simulink model "front_observer"  (R2025b)
settings: Solver=VariableStepAuto  StartTime=0.0  StopTime=60  RelTol=1e-3
undefined symbols (not defined in the file): A, B, C, L
settings Model: Creator=lilkiddy  LastModifiedBy=lilkiddy

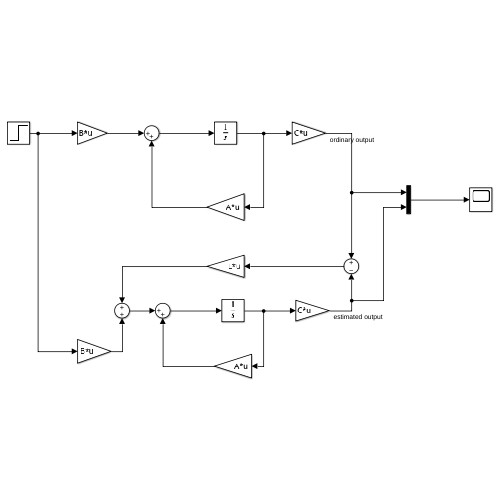
[thumbnail: Simulink's stored preview of the top-level diagram]
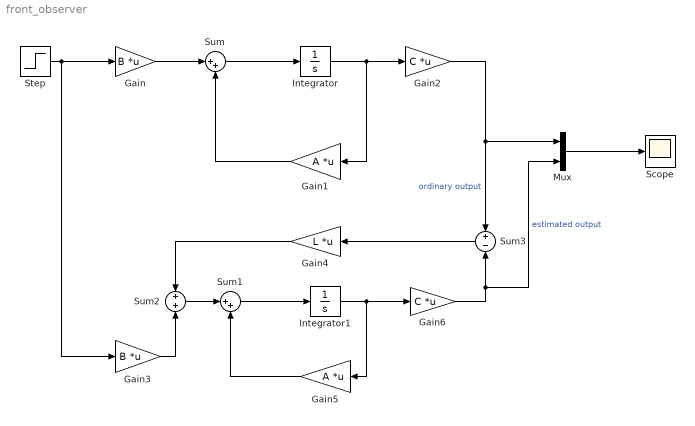
== system front_observer ==
  Gain : Gain  Gain=B  Multiplication=Matrix(K*u)
  Gain1 : Gain  Gain=A  Multiplication=Matrix(K*u)
  Gain2 : Gain  Gain=C  Multiplication=Matrix(K*u)
  Gain3 : Gain  Gain=B  Multiplication=Matrix(K*u)
  Gain4 : Gain  Gain=L  Multiplication=Matrix(K*u)
  Gain5 : Gain  Gain=A  Multiplication=Matrix(K*u)
  Gain6 : Gain  Gain=C  Multiplication=Matrix(K*u)
  Integrator : Integrator
  Integrator1 : Integrator
  Mux : Mux  Inputs=2
  Scope : Scope
      settings: ActiveDisplayYMinimum=-0.17957494978655622  ActiveDisplayYMaximum=1.6161745480790062  YLabel=displacement
  Step : Step  SampleTime=0
  Sum : Sum  Inputs=|++
  Sum1 : Sum  Inputs=|++
  Sum2 : Sum  Inputs=+|+
  Sum3 : Sum  Inputs=+|-
  wires:
  Step/1 -> Gain3/1, Gain/1
  Gain/1 -> Sum/1
  Sum/1 -> Integrator/1
  Gain1/1 -> Sum/2
  Integrator/1 -> Gain1/1, Gain2/1
  Gain2/1 -> Mux/1, Sum3/1  "ordinary output"
  Mux/1 -> Scope/1
  Sum2/1 -> Sum1/1
  Gain3/1 -> Sum2/2
  Gain4/1 -> Sum2/1
  Sum1/1 -> Integrator1/1
  Gain5/1 -> Sum1/2
  Integrator1/1 -> Gain5/1, Gain6/1
  Gain6/1 -> Mux/2, Sum3/2  "estimated output"
  Sum3/1 -> Gain4/1
